simulink model "Assgn3"  (R2021a)
settings: Solver=VariableStepAuto  StartTime=0.0  StopTime=10.0  RelTol=1e-3
values from neighbouring files (symbols this model uses):
  A1 = A-B*K    [Assgn3.m]
  B = [0;0;1/mc;1/(L*mc)]    [Assgn3.m]
settings Model: Creator=shrutidalal  LastModifiedBy=shrutidalal

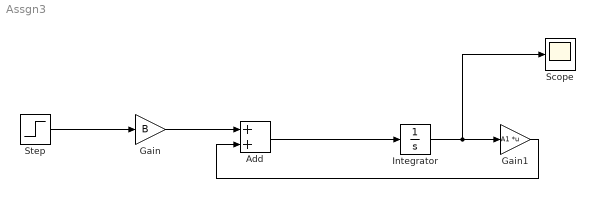
== system Assgn3 ==
  Add : Sum
  Gain : Gain  Gain=B
  Gain1 : Gain  Gain=A1  Multiplication=Matrix(K*u)
  Integrator : Integrator
  Scope : Scope
  Step : Step  SampleTime=0
  wires:
  Step/1 -> Gain/1
  Gain/1 -> Add/1
  Add/1 -> Integrator/1
  Integrator/1 -> Scope/1, Gain1/1
  Gain1/1 -> Add/2
